simulink model "dx_hand_model_rai3"  (R2017b)
settings: Solver=ode3  StartTime=0.0  StopTime=inf  FixedStep=0.01  RelTol=1e-3  EnableMultiTasking=on
InitFcn:
  | cutFreq = 0.1; % T
  | sampleTime = 0.01;
  | filt = tf(1,[cutFreq 1]);
  | filt = c2d(filt,sampleTime);
  | 
  | cutFreq2 = 1;
  | filt2 = tf(1,[cutFreq2 1]);
  | filt2 = c2d(filt2,sampleTime);
  | 
  | update_param = 2;
  | 
  | ampliFactor = 1.60;
  | ampliFactorMiddle = 2.00;
  | ampliFactorDistal = 1;
  | 
  | % Set Hand Address
  | RightHandAddress = '10.24.4.91';
  | Verosim = '10.100.39.22'
  | LeftHandAddress = '10.24.4.90'
  | 
  | max_force = 12; % Newton
model workspace (MAT data in the model file):
  SL_ROS_VariableLengthArrays_MaxSizes : struct (value not decoded)
libraries: robotlib x134, simulink_extras x28, simulink x16, dspnetwork x5, etargetslib x4
(part 4 of 19)

== system dx_hand_model_rai3/Send to Schunk/Signal Conditioning/Subsystem1 ==
  in_dis_in : Inport
  in_prox_in : Inport  Port=2
  Constant : Constant  Value=0  OutDataTypeStr=single
  Get Parameter3 : robotlib/Get Parameter  SourceLibraryInfo=This block requires Robotics System Toolbox  ParameterSource=Specify your own  ParameterName=/hand_exo/index/enable  ParameterType=double  ParameterMaxArrayLength=16  ParameterInitialValue=1.0  SampleTime=update_param  ShowErrorCodeOutput=on  ModelName=dx_hand_model_rai3  BlockId=ParamGet_dx_hand_model_rai3_2736
      settings: SourceProductName=Robotics System Toolbox  SourceProductBaseCode=RO
  Rate Transition : RateTransition
  Switch : Switch  Criteria=u2 > Threshold
  Switch1 : Switch  Criteria=u2 > Threshold
  in_dis_o : Outport
  in_prox_o : Outport  Port=2
  wires:
  Get Parameter3/1 -> Rate Transition/1
  Constant/1 -> Switch1/3, Switch/3
  in_dis_in/1 -> Switch1/1
  Switch1/1 -> in_dis_o/1
  Switch/1 -> in_prox_o/1
  Rate Transition/1 -> Switch1/2, Switch/2
  in_prox_in/1 -> Switch/1

== system dx_hand_model_rai3/Send to Schunk/Signal Conditioning/Subsystem2 ==
  m_dis_in : Inport
  m_prox_in : Inport  Port=2
  Constant : Constant  Value=0  OutDataTypeStr=single
  Display : Display
  Get Parameter3 : robotlib/Get Parameter  SourceLibraryInfo=This block requires Robotics System Toolbox  ParameterSource=Specify your own  ParameterName=/hand_exo/middle/enable  ParameterType=double  ParameterMaxArrayLength=16  ParameterInitialValue=1.0  SampleTime=update_param  ShowErrorCodeOutput=on  ModelName=dx_hand_model_rai3  BlockId=ParamGet_dx_hand_model_rai3_2745
      settings: SourceProductName=Robotics System Toolbox  SourceProductBaseCode=RO
  Rate Transition : RateTransition
  Switch : Switch  Criteria=u2 > Threshold
  Switch1 : Switch  Criteria=u2 > Threshold
  m_dis_o : Outport
  m_prox_o : Outport  Port=2
  wires:
  Get Parameter3/1 -> Rate Transition/1
  Constant/1 -> Switch1/3, Switch/3
  m_dis_in/1 -> Display/1, Switch1/1
  m_prox_in/1 -> Switch/1
  Switch1/1 -> m_dis_o/1
  Switch/1 -> m_prox_o/1
  Rate Transition/1 -> Switch1/2, Switch/2

== system dx_hand_model_rai3/Send to Schunk/Signal Conditioning/Subsystem3 ==
  r_in : Inport
  Constant : Constant  Value=0.0  OutDataTypeStr=single
  Get Parameter3 : robotlib/Get Parameter  SourceLibraryInfo=This block requires Robotics System Toolbox  ParameterSource=Specify your own  ParameterName=/hand_exo/ring/enable  ParameterType=double  ParameterMaxArrayLength=16  ParameterInitialValue=-1.0  SampleTime=update_param  ShowErrorCodeOutput=on  ModelName=dx_hand_model_rai3  BlockId=ParamGet_dx_hand_model_rai3_2754
      settings: SourceProductName=Robotics System Toolbox  SourceProductBaseCode=RO
  Rate Transition : RateTransition
  Switch1 : Switch  Criteria=u2 > Threshold
  r_o : Outport
  wires:
  Get Parameter3/1 -> Rate Transition/1
  Constant/1 -> Switch1/3
  r_in/1 -> Switch1/1
  Switch1/1 -> r_o/1
  Rate Transition/1 -> Switch1/2

== system dx_hand_model_rai3/Send to Schunk/Signal Conditioning/Subsystem4 ==
  p_in : Inport
  Constant : Constant  Value=0.0  OutDataTypeStr=single
  Get Parameter3 : robotlib/Get Parameter  SourceLibraryInfo=This block requires Robotics System Toolbox  ParameterSource=Specify your own  ParameterName=/hand_exo/pinky/enable  ParameterType=double  ParameterMaxArrayLength=16  ParameterInitialValue=-1.0  SampleTime=update_param  ShowErrorCodeOutput=on  ModelName=dx_hand_model_rai3  BlockId=ParamGet_dx_hand_model_rai3_2762
      settings: SourceProductName=Robotics System Toolbox  SourceProductBaseCode=RO
  Rate Transition : RateTransition
  Switch1 : Switch  Criteria=u2 > Threshold
  p_o : Outport
  wires:
  Get Parameter3/1 -> Rate Transition/1
  Constant/1 -> Switch1/3
  p_in/1 -> Switch1/1
  Switch1/1 -> p_o/1
  Rate Transition/1 -> Switch1/2

== system dx_hand_model_rai3/Send to Schunk/Signal Conditioning/Subsystem5 ==
  s_in : Inport
  Constant : Constant  Value=0.20  OutDataTypeStr=single
  Get Parameter3 : robotlib/Get Parameter  SourceLibraryInfo=This block requires Robotics System Toolbox  ParameterSource=Specify your own  ParameterName=/hand_exo/spread/enable  ParameterType=double  ParameterMaxArrayLength=16  ParameterInitialValue=-1.0  SampleTime=update_param  ShowErrorCodeOutput=on  ModelName=dx_hand_model_rai3  BlockId=ParamGet_dx_hand_model_rai3_2768
      settings: SourceProductName=Robotics System Toolbox  SourceProductBaseCode=RO
  Rate Transition : RateTransition
  Switch1 : Switch  Criteria=u2 > Threshold
  s_o : Outport
  wires:
  Get Parameter3/1 -> Rate Transition/1
  Constant/1 -> Switch1/3
  s_in/1 -> Switch1/1
  Switch1/1 -> s_o/1
  Rate Transition/1 -> Switch1/2

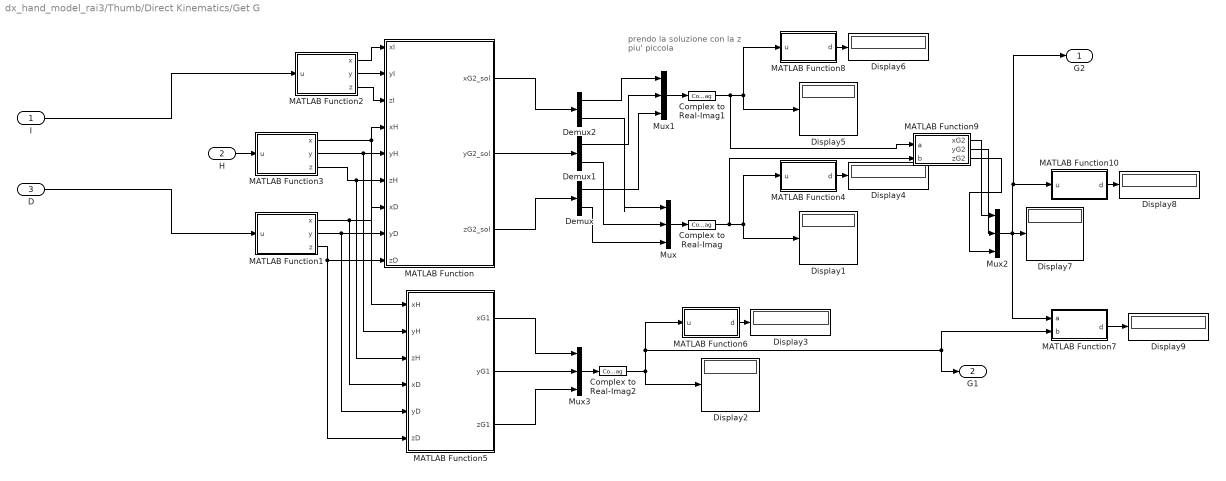
== system dx_hand_model_rai3/Thumb/Direct Kinematics/Get G ==
  note: prendo la soluzione
      | con la z piu' piccola
  I : Inport
  H : Inport  Port=2
  D : Inport  Port=3
  Complex to Real-Imag : ComplexToRealImag  Output=Real
  Complex to Real-Imag1 : ComplexToRealImag  Output=Real
  Complex to Real-Imag2 : ComplexToRealImag  Output=Real
  Demux : Demux  Outputs=2
  Demux1 : Demux  Outputs=2
  Demux2 : Demux  Outputs=2
  Display{1..9} (9 alike) : Display
  MATLAB Function : MATLAB Function  TreatAsAtomicUnit=on
  MATLAB Function1 : MATLAB Function  TreatAsAtomicUnit=on
  MATLAB Function10 : MATLAB Function  TreatAsAtomicUnit=on
  MATLAB Function2 : MATLAB Function  TreatAsAtomicUnit=on
  MATLAB Function3 : MATLAB Function  TreatAsAtomicUnit=on
  MATLAB Function4 : MATLAB Function  TreatAsAtomicUnit=on
  MATLAB Function5 : MATLAB Function  TreatAsAtomicUnit=on
  MATLAB Function6 : MATLAB Function  TreatAsAtomicUnit=on
  MATLAB Function7 : MATLAB Function  TreatAsAtomicUnit=on
  MATLAB Function8 : MATLAB Function  TreatAsAtomicUnit=on
  MATLAB Function9 : MATLAB Function  TreatAsAtomicUnit=on
  Mux{,1..3} (4 alike) : Mux  Inputs=3
  G2 : Outport
  G1 : Outport  Port=2
  wires:
  MATLAB Function1/2(y) -> MATLAB Function/8(yD), MATLAB Function5/5(yD)
  H/1 -> MATLAB Function3/1(u)
  MATLAB Function3/1(x) -> MATLAB Function5/1(xH), MATLAB Function/4(xH)
  MATLAB Function2/1(x) -> MATLAB Function/1(xI)
  D/1 -> MATLAB Function1/1(u)
  MATLAB Function/1(xG2_sol) -> Demux2/1
  Complex to Real-Imag1/1 -> MATLAB Function9/1(a), Display5/1, MATLAB Function8/1(u)
  Demux/2 -> Mux/3
  MATLAB Function10/1(d) -> Display8/1
  MATLAB Function/3(zG2_sol) -> Demux/1
  MATLAB Function2/3(z) -> MATLAB Function/3(zI)
  MATLAB Function2/2(y) -> MATLAB Function/2(yI)
  MATLAB Function9/3(zG2) -> Mux2/3
  Demux2/1 -> Mux1/1
  MATLAB Function1/3(z) -> MATLAB Function5/6(zD), MATLAB Function/9(zD)
  MATLAB Function9/1(xG2) -> Mux2/1
  Demux1/1 -> Mux1/2
  MATLAB Function1/1(x) -> MATLAB Function/7(xD), MATLAB Function5/4(xD)
  Complex to Real-Imag/1 -> MATLAB Function9/2(b), Display1/1, MATLAB Function4/1(u)
  Demux2/2 -> Mux/1
  MATLAB Function9/2(yG2) -> Mux2/2
  I/1 -> MATLAB Function2/1(u)
  Demux/1 -> Mux1/3
  Mux1/1 -> Complex to Real-Imag1/1
  Mux/1 -> Complex to Real-Imag/1
  MATLAB Function3/2(y) -> MATLAB Function5/2(yH), MATLAB Function/5(yH)
  MATLAB Function4/1(d) -> Display4/1
  MATLAB Function3/3(z) -> MATLAB Function/6(zH), MATLAB Function5/3(zH)
  Demux1/2 -> Mux/2
  MATLAB Function/2(yG2_sol) -> Demux1/1
  MATLAB Function8/1(d) -> Display6/1
  Mux3/1 -> Complex to Real-Imag2/1
  MATLAB Function5/2(yG1) -> Mux3/2
  MATLAB Function5/1(xG1) -> Mux3/1
  MATLAB Function5/3(zG1) -> Mux3/3
  MATLAB Function6/1(d) -> Display3/1
  Complex to Real-Imag2/1 -> Display2/1, G1/1, MATLAB Function7/2(b), MATLAB Function6/1(u)
  Mux2/1 -> MATLAB Function7/1(a), G2/1, MATLAB Function10/1(u), Display7/1
  MATLAB Function7/1(d) -> Display9/1

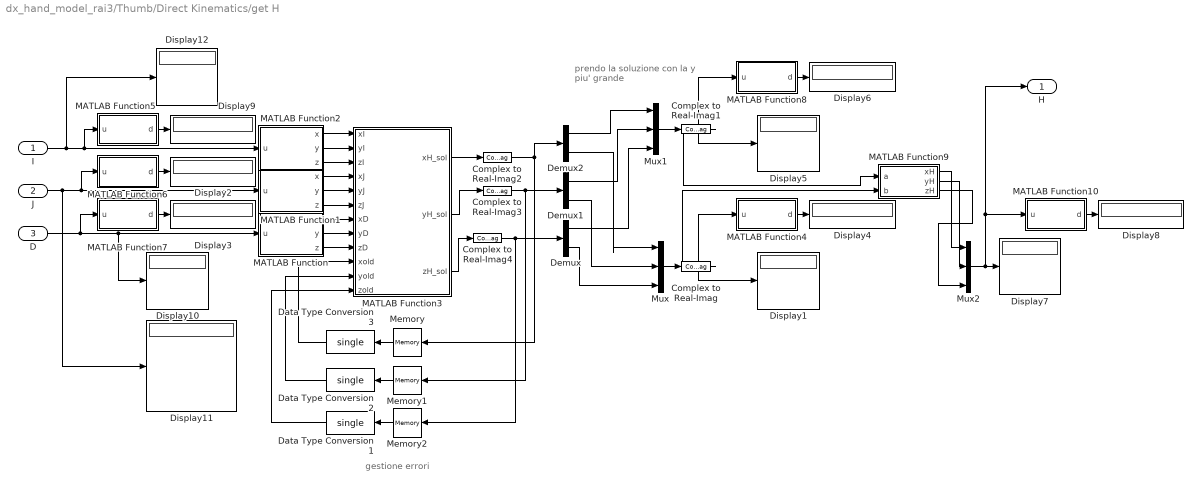
== system dx_hand_model_rai3/Thumb/Direct Kinematics/get H ==
  note: prendo la soluzione
      | con la y piu' grande
  note: gestione errori
  I : Inport
  J : Inport  Port=2
  D : Inport  Port=3
  Complex to Real-Imag{,1..4} (5 alike) : ComplexToRealImag  Output=Real
  Data Type Conversion1 : DataTypeConversion  OutDataTypeStr=single
  Data Type Conversion2 : DataTypeConversion  OutDataTypeStr=single
  Data Type Conversion3 : DataTypeConversion  OutDataTypeStr=single
  Demux : Demux  Outputs=2
  Demux1 : Demux  Outputs=2
  Demux2 : Demux  Outputs=2
  Display{1..12} (12 alike) : Display
  MATLAB Function : MATLAB Function  TreatAsAtomicUnit=on
  MATLAB Function1 : MATLAB Function  TreatAsAtomicUnit=on
  MATLAB Function10 : MATLAB Function  TreatAsAtomicUnit=on
  MATLAB Function2 : MATLAB Function  TreatAsAtomicUnit=on
  MATLAB Function3 : MATLAB Function  TreatAsAtomicUnit=on
  MATLAB Function4 : MATLAB Function  TreatAsAtomicUnit=on
  MATLAB Function5 : MATLAB Function  TreatAsAtomicUnit=on
  MATLAB Function6 : MATLAB Function  TreatAsAtomicUnit=on
  MATLAB Function7 : MATLAB Function  TreatAsAtomicUnit=on
  MATLAB Function8 : MATLAB Function  TreatAsAtomicUnit=on
  MATLAB Function9 : MATLAB Function  TreatAsAtomicUnit=on
  Memory : Memory  InitialCondition=[0,0]
  Memory1 : Memory  InitialCondition=[0,0]
  Memory2 : Memory  InitialCondition=[0,0]
  Mux : Mux  Inputs=3
  Mux1 : Mux  Inputs=3
  Mux2 : Mux  Inputs=3
  H : Outport
  wires:
  MATLAB Function3/1(xH_sol) -> Complex to Real-Imag2/1
  MATLAB Function3/2(yH_sol) -> Complex to Real-Imag3/1
  MATLAB Function9/2(yH) -> Mux2/2
  MATLAB Function9/1(xH) -> Mux2/1
  MATLAB Function4/1(d) -> Display4/1
  Mux2/1 -> H/1, MATLAB Function10/1(u), Display7/1
  Demux2/2 -> Mux/1
  MATLAB Function8/1(d) -> Display6/1
  MATLAB Function6/1(d) -> Display2/1
  MATLAB Function5/1(d) -> Display9/1
  MATLAB Function9/3(zH) -> Mux2/3
  Demux/2 -> Mux/3
  Complex to Real-Imag1/1 -> MATLAB Function9/1(a), Display5/1, MATLAB Function8/1(u)
  Complex to Real-Imag/1 -> MATLAB Function9/2(b), Display1/1, MATLAB Function4/1(u)
  MATLAB Function7/1(d) -> Display3/1
  Demux1/1 -> Mux1/2
  Mux/1 -> Complex to Real-Imag/1
  MATLAB Function10/1(d) -> Display8/1
  Demux2/1 -> Mux1/1
  Demux/1 -> Mux1/3
  MATLAB Function2/2(y) -> MATLAB Function3/2(yI)
  MATLAB Function2/1(x) -> MATLAB Function3/1(xI)
  Demux1/2 -> Mux/2
  MATLAB Function/1(x) -> MATLAB Function3/7(xD)
  D/1 -> MATLAB Function7/1(u), Display10/1, MATLAB Function/1(u)
  MATLAB Function/3(z) -> MATLAB Function3/9(zD)
  MATLAB Function/2(y) -> MATLAB Function3/8(yD)
  MATLAB Function1/1(x) -> MATLAB Function3/4(xJ)
  MATLAB Function1/3(z) -> MATLAB Function3/6(zJ)
  I/1 -> Display12/1, MATLAB Function5/1(u), MATLAB Function2/1(u)
  J/1 -> Display11/1, MATLAB Function6/1(u), MATLAB Function1/1(u)
  MATLAB Function1/2(y) -> MATLAB Function3/5(yJ)
  MATLAB Function2/3(z) -> MATLAB Function3/3(zI)
  Mux1/1 -> Complex to Real-Imag1/1
  MATLAB Function3/3(zH_sol) -> Complex to Real-Imag4/1
  Memory/1 -> Data Type Conversion3/1
  Memory1/1 -> Data Type Conversion2/1
  Memory2/1 -> Data Type Conversion1/1
  Data Type Conversion1/1 -> MATLAB Function3/12(zold)
  Data Type Conversion2/1 -> MATLAB Function3/11(yold)
  Data Type Conversion3/1 -> MATLAB Function3/10(xold)
  Complex to Real-Imag2/1 -> Demux2/1, Memory/1
  Complex to Real-Imag3/1 -> Memory1/1, Demux1/1
  Complex to Real-Imag4/1 -> Memory2/1, Demux/1

== system dx_hand_model_rai3/Thumb/Force Feedback/Active ==
  in : Inport
  Constant : Constant  Value=0  OutDataTypeStr=single
  Data Type Conversion1 : DataTypeConversion  OutDataTypeStr=single
  Get Parameter3 : robotlib/Get Parameter  SourceLibraryInfo=This block requires Robotics System Toolbox  ParameterSource=Specify your own  ParameterName=/hand_exo/thumb/modes/ff_active  ParameterType=double  ParameterMaxArrayLength=16  ParameterInitialValue=1.0  SampleTime=update_param  ShowErrorCodeOutput=off  ModelName=dx_hand_model_rai3  BlockId=ParamGet_dx_hand_model_rai3_4863
      settings: SourceProductName=Robotics System Toolbox  SourceProductBaseCode=RO
  Rate Transition : RateTransition
  Switch : Switch  Criteria=u2 > Threshold
  out : Outport
  wires:
  Switch/1 -> out/1
  Data Type Conversion1/1 -> Switch/2
  Rate Transition/1 -> Data Type Conversion1/1
  Get Parameter3/1 -> Rate Transition/1
  in/1 -> Switch/1
  Constant/1 -> Switch/3

== system dx_hand_model_rai3/Thumb/Force Feedback/g1 ==
  in : Inport
  Data Type Conversion1 : DataTypeConversion  OutDataTypeStr=single
  Get Parameter3 : robotlib/Get Parameter  SourceLibraryInfo=This block requires Robotics System Toolbox  ParameterSource=Specify your own  ParameterName=/hand_exo/thumb/gain/g1  ParameterType=double  ParameterMaxArrayLength=16  ParameterInitialValue=3.5  SampleTime=update_param  ShowErrorCodeOutput=on  ModelName=dx_hand_model_rai3  BlockId=ParamGet_dx_hand_model_rai3_3828
      settings: SourceProductName=Robotics System Toolbox  SourceProductBaseCode=RO
  Product : Product
  Rate Transition : RateTransition
  "out " : Outport
  wires:
  Get Parameter3/1 -> Rate Transition/1
  Rate Transition/1 -> Data Type Conversion1/1
  Data Type Conversion1/1 -> Product/2
  Product/1 -> "out "/1
  in/1 -> Product/1

== system dx_hand_model_rai3/Thumb/Get ADC Values/Angular Potentiometer 1 ==
  ADC : Inport
  Constant : Constant  Value=0  OutDataTypeStr=single
  Constant1 : Constant  Value=420  OutDataTypeStr=single
  Data Type Conversion1 : DataTypeConversion  OutDataTypeStr=single
  Data Type Conversion2 : DataTypeConversion  OutDataTypeStr=double
  Display : Display
  Display1 : Display
  Display2 : Display
  Gain Aggiustato : Gain  Gain=330*pi/(1024*180)
  Get Parameter3 : robotlib/Get Parameter  SourceLibraryInfo=This block requires Robotics System Toolbox  ParameterSource=Specify your own  ParameterName=/hand_exo/thumb/calibration/set1  ParameterType=double  ParameterMaxArrayLength=16  ParameterInitialValue=381  SampleTime=update_param  ShowErrorCodeOutput=on  ModelName=dx_hand_model_rai3  BlockId=ParamGet_dx_hand_model_rai3_2962
      settings: SourceProductName=Robotics System Toolbox  SourceProductBaseCode=RO
  Manual Switch : ManualSwitch
  Radians to Degrees : simulink_extras/Transformations/Radians to Degrees
  Rate Transition : RateTransition
  Set Parameter : robotlib/Set Parameter  SourceLibraryInfo=This block requires Robotics System Toolbox  ParameterSource=Specify your own  ParameterName=/hand_exo/thumb/calibration/get1  ParameterType=double  ModelName=dx_hand_model_rai3  BlockId=ParamSet_dx_hand_model_rai3_2966
      settings: SourceProductName=Robotics System Toolbox  SourceProductBaseCode=RO
  Sum1 : Sum  Inputs=|+-
  Sum2 : Sum  Inputs=|+-
  Deg : Outport
  Rad : Outport  Port=2
  wires:
  ADC/1 -> Data Type Conversion2/1, Sum2/1
  Radians to Degrees/1 -> Display1/1, Deg/1
  Gain Aggiustato/1 -> Display/1, Sum1/1
  Sum1/1 -> Radians to Degrees/1, Rad/1
  Constant/1 -> Sum1/2
  Sum2/1 -> Gain Aggiustato/1
  Get Parameter3/1 -> Rate Transition/1
  Data Type Conversion2/1 -> Set Parameter/1, Display2/1
  Rate Transition/1 -> Data Type Conversion1/1
  Data Type Conversion1/1 -> Manual Switch/1
  Manual Switch/1 -> Sum2/2
  Constant1/1 -> Manual Switch/2

== system dx_hand_model_rai3/Thumb/Get ADC Values/Angular Potentiometer 2 ==
  ADC : Inport
  Constant : Constant  Value=0  OutDataTypeStr=single
  Constant1 : Constant  Value=529  OutDataTypeStr=single
  Data Type Conversion1 : DataTypeConversion  OutDataTypeStr=single
  Data Type Conversion2 : DataTypeConversion  OutDataTypeStr=double
  Display : Display
  Display1 : Display
  Display2 : Display
  Gain Aggiustato : Gain  Gain=330*pi/(1024*180)
  Get Parameter3 : robotlib/Get Parameter  SourceLibraryInfo=This block requires Robotics System Toolbox  ParameterSource=Specify your own  ParameterName=/hand_exo/thumb/calibration/set2  ParameterType=double  ParameterMaxArrayLength=16  ParameterInitialValue=529  SampleTime=update_param  ShowErrorCodeOutput=on  ModelName=dx_hand_model_rai3  BlockId=ParamGet_dx_hand_model_rai3_3019
      settings: SourceProductName=Robotics System Toolbox  SourceProductBaseCode=RO
  Manual Switch : ManualSwitch
  Radians to Degrees : simulink_extras/Transformations/Radians to Degrees
  Rate Transition : RateTransition
  Set Parameter : robotlib/Set Parameter  SourceLibraryInfo=This block requires Robotics System Toolbox  ParameterSource=Specify your own  ParameterName=/hand_exo/thumb/calibration/get2  ParameterType=double  ModelName=dx_hand_model_rai3  BlockId=ParamSet_dx_hand_model_rai3_3023
      settings: SourceProductName=Robotics System Toolbox  SourceProductBaseCode=RO
  Sum1 : Sum  Inputs=|+-
  Sum2 : Sum  Inputs=|+-
  Deg : Outport
  Rad : Outport  Port=2
  wires:
  ADC/1 -> Data Type Conversion2/1, Sum2/1
  Radians to Degrees/1 -> Display1/1, Deg/1
  Gain Aggiustato/1 -> Display/1, Sum1/1
  Sum1/1 -> Radians to Degrees/1, Rad/1
  Constant/1 -> Sum1/2
  Sum2/1 -> Gain Aggiustato/1
  Get Parameter3/1 -> Rate Transition/1
  Data Type Conversion2/1 -> Set Parameter/1, Display2/1
  Rate Transition/1 -> Data Type Conversion1/1
  Data Type Conversion1/1 -> Manual Switch/1
  Manual Switch/1 -> Sum2/2
  Constant1/1 -> Manual Switch/2

== system dx_hand_model_rai3/Thumb/Get ADC Values/Angular Potentiometer 3 ==
  ADC : Inport
  Constant : Constant  Value=0  OutDataTypeStr=single
  Constant1 : Constant  Value=576  OutDataTypeStr=single
  Data Type Conversion1 : DataTypeConversion  OutDataTypeStr=single
  Data Type Conversion2 : DataTypeConversion  OutDataTypeStr=double
  Display : Display
  Display1 : Display
  Display2 : Display
  Gain Aggiustato : Gain  Gain=330*pi/(1024*180)
  Get Parameter3 : robotlib/Get Parameter  SourceLibraryInfo=This block requires Robotics System Toolbox  ParameterSource=Specify your own  ParameterName=/hand_exo/thumb/calibration/set3  ParameterType=double  ParameterMaxArrayLength=16  ParameterInitialValue=576  SampleTime=update_param  ShowErrorCodeOutput=on  ModelName=dx_hand_model_rai3  BlockId=ParamGet_dx_hand_model_rai3_3038
      settings: SourceProductName=Robotics System Toolbox  SourceProductBaseCode=RO
  Manual Switch : ManualSwitch
  Radians to Degrees : simulink_extras/Transformations/Radians to Degrees
  Rate Transition : RateTransition
  Set Parameter : robotlib/Set Parameter  SourceLibraryInfo=This block requires Robotics System Toolbox  ParameterSource=Specify your own  ParameterName=/hand_exo/thumb/calibration/get3  ParameterType=double  ModelName=dx_hand_model_rai3  BlockId=ParamSet_dx_hand_model_rai3_3042
      settings: SourceProductName=Robotics System Toolbox  SourceProductBaseCode=RO
  Sum1 : Sum  Inputs=|+-
  Sum2 : Sum  Inputs=|+-
  Deg : Outport
  Rad : Outport  Port=2
  wires:
  ADC/1 -> Data Type Conversion2/1, Sum2/1
  Radians to Degrees/1 -> Display1/1, Deg/1
  Gain Aggiustato/1 -> Display/1, Sum1/1
  Sum1/1 -> Radians to Degrees/1, Rad/1
  Constant/1 -> Sum1/2
  Sum2/1 -> Gain Aggiustato/1
  Get Parameter3/1 -> Rate Transition/1
  Data Type Conversion2/1 -> Set Parameter/1, Display2/1
  Rate Transition/1 -> Data Type Conversion1/1
  Data Type Conversion1/1 -> Manual Switch/1
  Manual Switch/1 -> Sum2/2
  Constant1/1 -> Manual Switch/2

== system dx_hand_model_rai3/Thumb/Get ADC Values/Angular Potentiometer 4 ==
  ADC : Inport
  Constant2 : Constant  Value=517  OutDataTypeStr=single
  Data Type Conversion1 : DataTypeConversion  OutDataTypeStr=single
  Data Type Conversion2 : DataTypeConversion  OutDataTypeStr=double
  Display : Display
  Display1 : Display
  Display3 : Display
  Gain Aggiustato : Gain  Gain=330*pi/(1024*180)
  Get Parameter3 : robotlib/Get Parameter  SourceLibraryInfo=This block requires Robotics System Toolbox  ParameterSource=Specify your own  ParameterName=/hand_exo/thumb/calibration/set4  ParameterType=double  ParameterMaxArrayLength=16  ParameterInitialValue=517.0  SampleTime=update_param  ShowErrorCodeOutput=on  ModelName=dx_hand_model_rai3  BlockId=ParamGet_dx_hand_model_rai3_4259
      settings: SourceProductName=Robotics System Toolbox  SourceProductBaseCode=RO
  Manual Switch : ManualSwitch
  Radians to Degrees : simulink_extras/Transformations/Radians to Degrees
  Rate Transition : RateTransition
  Set Parameter : robotlib/Set Parameter  SourceLibraryInfo=This block requires Robotics System Toolbox  ParameterSource=Specify your own  ParameterName=/hand_exo/thumb/calibration/get4  ParameterType=double  ModelName=dx_hand_model_rai3  BlockId=ParamSet_dx_hand_model_rai3_4262
      settings: SourceProductName=Robotics System Toolbox  SourceProductBaseCode=RO
  Sign : Gain  Gain=-1
  Sum2 : Sum  Inputs=|+-
  Deg : Outport
  Rad : Outport  Port=2
  wires:
  Radians to Degrees/1 -> Display1/1, Deg/1
  ADC/1 -> Sum2/1, Data Type Conversion2/1
  Gain Aggiustato/1 -> Sign/1, Display/1
  Sign/1 -> Radians to Degrees/1, Rad/1
  Sum2/1 -> Gain Aggiustato/1
  Manual Switch/1 -> Sum2/2
  Get Parameter3/1 -> Rate Transition/1
  Data Type Conversion2/1 -> Set Parameter/1, Display3/1
  Rate Transition/1 -> Data Type Conversion1/1
  Data Type Conversion1/1 -> Manual Switch/1
  Constant2/1 -> Manual Switch/2

== system dx_hand_model_rai3/Thumb/Get ADC Values/Angular Potentiometer 5 ==
  ADC : Inport
  Constant2 : Constant  Value=579  OutDataTypeStr=single
  Data Type Conversion1 : DataTypeConversion  OutDataTypeStr=single
  Data Type Conversion2 : DataTypeConversion  OutDataTypeStr=double
  Display : Display
  Display1 : Display
  Display3 : Display
  Gain Aggiustato : Gain  Gain=330*pi/(1024*180)
  Get Parameter3 : robotlib/Get Parameter  SourceLibraryInfo=This block requires Robotics System Toolbox  ParameterSource=Specify your own  ParameterName=/hand_exo/thumb/calibration/set5  ParameterType=double  ParameterMaxArrayLength=16  ParameterInitialValue=579.0  SampleTime=update_param  ShowErrorCodeOutput=on  ModelName=dx_hand_model_rai3  BlockId=ParamGet_dx_hand_model_rai3_4267
      settings: SourceProductName=Robotics System Toolbox  SourceProductBaseCode=RO
  Manual Switch : ManualSwitch
  Radians to Degrees : simulink_extras/Transformations/Radians to Degrees
  Rate Transition : RateTransition
  Set Parameter : robotlib/Set Parameter  SourceLibraryInfo=This block requires Robotics System Toolbox  ParameterSource=Specify your own  ParameterName=/hand_exo/thumb/calibration/get5  ParameterType=double  ModelName=dx_hand_model_rai3  BlockId=ParamSet_dx_hand_model_rai3_4270
      settings: SourceProductName=Robotics System Toolbox  SourceProductBaseCode=RO
  Sign : Gain
  Sum2 : Sum  Inputs=|+-
  Deg : Outport
  Rad : Outport  Port=2
  wires:
  Radians to Degrees/1 -> Display1/1, Deg/1
  Gain Aggiustato/1 -> Sign/1, Display/1
  Sign/1 -> Radians to Degrees/1, Rad/1
  Sum2/1 -> Gain Aggiustato/1
  ADC/1 -> Data Type Conversion2/1, Sum2/1
  Manual Switch/1 -> Sum2/2
  Get Parameter3/1 -> Rate Transition/1
  Constant2/1 -> Manual Switch/2
  Data Type Conversion2/1 -> Set Parameter/1, Display3/1
  Rate Transition/1 -> Data Type Conversion1/1
  Data Type Conversion1/1 -> Manual Switch/1

== system dx_hand_model_rai3/Thumb/Get_from_ROS_param/Subsystem ==
  In1 : Inport
  Data Type Conversion1 : DataTypeConversion  OutDataTypeStr=single
  Rate Transition : RateTransition  InitialCondition=-10.0
  Out1 : Outport
  wires:
  Data Type Conversion1/1 -> Out1/1
  In1/1 -> Rate Transition/1
  Rate Transition/1 -> Data Type Conversion1/1

== system dx_hand_model_rai3/Thumb/Get_from_ROS_param/Subsystem1 ==
  In1 : Inport
  Data Type Conversion1 : DataTypeConversion  OutDataTypeStr=single
  Rate Transition : RateTransition  InitialCondition=0.0
  Out1 : Outport
  wires:
  Data Type Conversion1/1 -> Out1/1
  In1/1 -> Rate Transition/1
  Rate Transition/1 -> Data Type Conversion1/1

== system dx_hand_model_rai3/Thumb/Get_from_ROS_param/Subsystem2 ==
  In1 : Inport
  Data Type Conversion1 : DataTypeConversion  OutDataTypeStr=single
  Rate Transition : RateTransition  InitialCondition=-32.0
  Out1 : Outport
  wires:
  Data Type Conversion1/1 -> Out1/1
  In1/1 -> Rate Transition/1
  Rate Transition/1 -> Data Type Conversion1/1

== system dx_hand_model_rai3/Thumb/Get_from_ROS_param/Subsystem3 ==
  In1 : Inport
  Data Type Conversion1 : DataTypeConversion  OutDataTypeStr=single
  Rate Transition : RateTransition  InitialCondition=20.0
  Out1 : Outport
  wires:
  Data Type Conversion1/1 -> Out1/1
  In1/1 -> Rate Transition/1
  Rate Transition/1 -> Data Type Conversion1/1

== system dx_hand_model_rai3/Thumb/Get_from_ROS_param/Subsystem4 ==
  In1 : Inport
  Data Type Conversion1 : DataTypeConversion  OutDataTypeStr=single
  Rate Transition : RateTransition  InitialCondition=50.0
  Out1 : Outport
  wires:
  Data Type Conversion1/1 -> Out1/1
  In1/1 -> Rate Transition/1
  Rate Transition/1 -> Data Type Conversion1/1

== system dx_hand_model_rai3/Thumb/Get_from_ROS_param/Subsystem5 ==
  In1 : Inport
  Data Type Conversion1 : DataTypeConversion  OutDataTypeStr=single
  Rate Transition : RateTransition  InitialCondition=20.0
  Out1 : Outport
  wires:
  Data Type Conversion1/1 -> Out1/1
  In1/1 -> Rate Transition/1
  Rate Transition/1 -> Data Type Conversion1/1

== system dx_hand_model_rai3/Thumb/Get_from_ROS_param/Subsystem6 ==
  In1 : Inport
  Data Type Conversion1 : DataTypeConversion  OutDataTypeStr=single
  Rate Transition : RateTransition  InitialCondition=50.0
  Out1 : Outport
  wires:
  Data Type Conversion1/1 -> Out1/1
  In1/1 -> Rate Transition/1
  Rate Transition/1 -> Data Type Conversion1/1

== system dx_hand_model_rai3/Thumb/Old Stuff/calibration ==
  In1 : Inport
  Constant2 : Constant  Value=540  OutDataTypeStr=single
  Constant3 : Constant  Value=540  OutDataTypeStr=single
  Display4 : Display
  Subsystem : Subsystem
  Sum2 : Sum  Inputs=|++
  Switch : Switch  Criteria=u2 > Threshold
  Out1 : Outport
  wires:
  [CalibrationSignal] -> Switch/2
  Subsystem/1(Out1) -> Switch/3
  Constant3/1 -> Sum2/1
  [CalibrationSignal] -> Subsystem/Enable
  Constant2/1 -> Switch/1
  Sum2/1 -> Display4/1, Subsystem/1(In1)
  In1/1 -> Sum2/2
  Switch/1 -> Out1/1

== system dx_hand_model_rai3/Thumb/Old Stuff/calibration1 ==
  In1 : Inport
  Subsystem1 : Subsystem
  Out1 : Outport
  wires:
  [CalibrationSignal] -> Subsystem1/Enable
  In1/1 -> Subsystem1/1(In1)
  Subsystem1/1(Out1) -> Out1/1

== system dx_hand_model_rai3/Thumb/Study Gravity Compensation/Subsystem2 ==
  In1 : Inport
  In2 : Inport  Port=2
  Enable : EnablePort
  Data Type Conversion1 : DataTypeConversion  OutDataTypeStr=double
  Mux : Mux  Inputs=2
  To File : ToFile  Filename=thumb_force.mat  MatrixName=forza_gravita
  wires:
  In1/1 -> Mux/1
  Mux/1 -> Data Type Conversion1/1
  In2/1 -> Mux/2
  Data Type Conversion1/1 -> To File/1

== system dx_hand_model_rai3/Thumb/ToSchunk/Subsystem ==
  Data Type Conversion1 : DataTypeConversion  OutDataTypeStr=single
  Get Parameter3 : robotlib/Get Parameter  SourceLibraryInfo=This block requires Robotics System Toolbox  ParameterSource=Specify your own  ParameterName=/hand_exo/thumb/offset/opp  ParameterType=double  ParameterMaxArrayLength=16  ParameterInitialValue=0.5  SampleTime=update_param  ShowErrorCodeOutput=on  ModelName=dx_hand_model_rai3  BlockId=ParamGet_dx_hand_model_rai3_3810
      settings: SourceProductName=Robotics System Toolbox  SourceProductBaseCode=RO
  Rate Transition : RateTransition
  offset : Outport
  wires:
  Get Parameter3/1 -> Rate Transition/1
  Rate Transition/1 -> Data Type Conversion1/1
  Data Type Conversion1/1 -> offset/1

== system dx_hand_model_rai3/Thumb/ToSchunk/Subsystem1 ==
  Data Type Conversion1 : DataTypeConversion  OutDataTypeStr=single
  Get Parameter3 : robotlib/Get Parameter  SourceLibraryInfo=This block requires Robotics System Toolbox  ParameterSource=Specify your own  ParameterName=/hand_exo/thumb/offset/flex  ParameterType=double  ParameterMaxArrayLength=16  ParameterInitialValue=5.0  SampleTime=update_param  ShowErrorCodeOutput=on  ModelName=dx_hand_model_rai3  BlockId=ParamGet_dx_hand_model_rai3_3817
      settings: SourceProductName=Robotics System Toolbox  SourceProductBaseCode=RO
  Rate Transition : RateTransition
  offset : Outport
  wires:
  Get Parameter3/1 -> Rate Transition/1
  Rate Transition/1 -> Data Type Conversion1/1
  Data Type Conversion1/1 -> offset/1

== system dx_hand_model_rai3/Get From Schunk/Get positions/Get Positions/Filter ==
  enable : Inport
  in : Inport  Port=2
  Filt 4 : DiscreteTransferFcn  Numerator=filt2.Numerator{1,1}  Denominator=filt2.Denominator{1,1}  SampleTime=0.01
  Switch : Switch  Criteria=u2 > Threshold
  out : Outport
  wires:
  in/1 -> Switch/3, Filt 4/1
  Switch/1 -> out/1
  Filt 4/1 -> Switch/1
  enable/1 -> Switch/2

== system dx_hand_model_rai3/Get From Schunk/Get positions/Get Positions/Filter1 ==
  enable : Inport
  in : Inport  Port=2
  Filt 4 : DiscreteTransferFcn  Numerator=filt2.Numerator{1,1}  Denominator=filt2.Denominator{1,1}  SampleTime=0.01
  Switch : Switch  Criteria=u2 > Threshold
  out : Outport
  wires:
  in/1 -> Switch/3, Filt 4/1
  Switch/1 -> out/1
  Filt 4/1 -> Switch/1
  enable/1 -> Switch/2

== system dx_hand_model_rai3/Get From Schunk/Get positions/Get Positions/Filter2 ==
  enable : Inport
  in : Inport  Port=2
  Filt 4 : DiscreteTransferFcn  Numerator=filt2.Numerator{1,1}  Denominator=filt2.Denominator{1,1}  SampleTime=0.01
  Switch : Switch  Criteria=u2 > Threshold
  out : Outport
  wires:
  in/1 -> Switch/3, Filt 4/1
  Switch/1 -> out/1
  Filt 4/1 -> Switch/1
  enable/1 -> Switch/2

== system dx_hand_model_rai3/Get From Schunk/Get positions/Get Positions/Filter3 ==
  enable : Inport
  in : Inport  Port=2
  Filt 4 : DiscreteTransferFcn  Numerator=filt2.Numerator{1,1}  Denominator=filt2.Denominator{1,1}  SampleTime=0.01
  Switch : Switch  Criteria=u2 > Threshold
  out : Outport
  wires:
  in/1 -> Switch/3, Filt 4/1
  Switch/1 -> out/1
  Filt 4/1 -> Switch/1
  enable/1 -> Switch/2

== system dx_hand_model_rai3/Get From Schunk/Get positions/Get Positions/Filter4 ==
  enable : Inport
  in : Inport  Port=2
  Filt 4 : DiscreteTransferFcn  Numerator=filt2.Numerator{1,1}  Denominator=filt2.Denominator{1,1}  SampleTime=0.01
  Switch : Switch  Criteria=u2 > Threshold
  out : Outport
  wires:
  in/1 -> Switch/3, Filt 4/1
  Switch/1 -> out/1
  Filt 4/1 -> Switch/1
  enable/1 -> Switch/2

== system dx_hand_model_rai3/Get From Schunk/Get positions/Get Positions/Filter5 ==
  enable : Inport
  in : Inport  Port=2
  Filt 4 : DiscreteTransferFcn  Numerator=filt2.Numerator{1,1}  Denominator=filt2.Denominator{1,1}  SampleTime=0.01
  Switch : Switch  Criteria=u2 > Threshold
  out : Outport
  wires:
  in/1 -> Switch/3, Filt 4/1
  Switch/1 -> out/1
  Filt 4/1 -> Switch/1
  enable/1 -> Switch/2

== system dx_hand_model_rai3/Index Finger/Force/Position Force Basic Architecture/pos_gains//dist ==
  pre_dist : Inport
  Constant : Constant  Value=10  OutDataTypeStr=single
  Data Type Conversion1 : DataTypeConversion  OutDataTypeStr=single
  Data Type Conversion2 : DataTypeConversion  OutDataTypeStr=single
  Get Parameter3 : robotlib/Get Parameter  SourceLibraryInfo=This block requires Robotics System Toolbox  ParameterSource=Specify your own  ParameterName=/hand_exo/index/f_gains/dist  ParameterType=double  ParameterMaxArrayLength=16  ParameterInitialValue=0.0  SampleTime=update_param  ShowErrorCodeOutput=on  ModelName=dx_hand_model_rai3  BlockId=ParamGet_dx_hand_model_rai3_3578
      settings: SourceProductName=Robotics System Toolbox  SourceProductBaseCode=RO
  Manual Switch : ManualSwitch
  Product : Product
  Rate Transition : RateTransition
  post_dist : Outport
  wires:
  Get Parameter3/1 -> Rate Transition/1
  pre_dist/1 -> Product/2
  Product/1 -> Data Type Conversion1/1
  Data Type Conversion1/1 -> post_dist/1
  Rate Transition/1 -> Data Type Conversion2/1
  Constant/1 -> Manual Switch/2
  Data Type Conversion2/1 -> Manual Switch/1
  Manual Switch/1 -> Product/1

== system dx_hand_model_rai3/Index Finger/Force/Position Force Basic Architecture/pos_gains//prox ==
  pre_prox : Inport
  Constant : Constant  Value=-15  OutDataTypeStr=single
  Data Type Conversion1 : DataTypeConversion  OutDataTypeStr=single
  Data Type Conversion2 : DataTypeConversion  OutDataTypeStr=single
  Get Parameter3 : robotlib/Get Parameter  SourceLibraryInfo=This block requires Robotics System Toolbox  ParameterSource=Specify your own  ParameterName=/hand_exo/index/f_gains/prox  ParameterType=double  ParameterMaxArrayLength=16  ParameterInitialValue=-15  SampleTime=update_param  ShowErrorCodeOutput=on  ModelName=dx_hand_model_rai3  BlockId=ParamGet_dx_hand_model_rai3_3588
      settings: SourceProductName=Robotics System Toolbox  SourceProductBaseCode=RO
  Manual Switch : ManualSwitch
  Product : Product
  Rate Transition : RateTransition
  post_prox : Outport
  wires:
  Get Parameter3/1 -> Rate Transition/1
  pre_prox/1 -> Product/2
  Product/1 -> Data Type Conversion1/1
  Data Type Conversion1/1 -> post_prox/1
  Rate Transition/1 -> Data Type Conversion2/1
  Data Type Conversion2/1 -> Manual Switch/1
  Manual Switch/1 -> Product/1
  Constant/1 -> Manual Switch/2

== system dx_hand_model_rai3/Index Finger/Pose Generator/Parametri Dito/Get_from_ROS_param ==
  Get Parameter : robotlib/Get Parameter  SourceLibraryInfo=This block requires Robotics System Toolbox  ParameterSource=Specify your own  ParameterName=/hand_exo/index/offx  ParameterType=double  ParameterMaxArrayLength=16  ParameterInitialValue=0.0  SampleTime=update_param  ShowErrorCodeOutput=on  ModelName=dx_hand_model_rai3  BlockId=ParamGet_dx_hand_model_rai3_2613
      settings: SourceProductName=Robotics System Toolbox  SourceProductBaseCode=RO
  Get Parameter1 : robotlib/Get Parameter  SourceLibraryInfo=This block requires Robotics System Toolbox  ParameterSource=Specify your own  ParameterName=/hand_exo/index/offy  ParameterType=double  ParameterMaxArrayLength=16  ParameterInitialValue=20.0  SampleTime=update_param  ShowErrorCodeOutput=on  ModelName=dx_hand_model_rai3  BlockId=ParamGet_dx_hand_model_rai3_2614
      settings: SourceProductName=Robotics System Toolbox  SourceProductBaseCode=RO
  Get Parameter2 : robotlib/Get Parameter  SourceLibraryInfo=This block requires Robotics System Toolbox  ParameterSource=Specify your own  ParameterName=/hand_exo/index/length  ParameterType=double  ParameterMaxArrayLength=16  ParameterInitialValue=44.0  SampleTime=update_param  ShowErrorCodeOutput=on  ModelName=dx_hand_model_rai3  BlockId=ParamGet_dx_hand_model_rai3_2615
      settings: SourceProductName=Robotics System Toolbox  SourceProductBaseCode=RO
  Get Parameter3 : robotlib/Get Parameter  SourceLibraryInfo=This block requires Robotics System Toolbox  ParameterSource=Specify your own  ParameterName=/hand_exo/index/s  ParameterType=double  ParameterMaxArrayLength=16  ParameterInitialValue=8.5  SampleTime=update_param  ShowErrorCodeOutput=on  ModelName=dx_hand_model_rai3  BlockId=ParamGet_dx_hand_model_rai3_2616
      settings: SourceProductName=Robotics System Toolbox  SourceProductBaseCode=RO
  Get Parameter4 : robotlib/Get Parameter  SourceLibraryInfo=This block requires Robotics System Toolbox  ParameterSource=Specify your own  ParameterName=/hand_exo/index/offa  ParameterType=double  ParameterMaxArrayLength=16  ParameterInitialValue=0  SampleTime=update_param  ShowErrorCodeOutput=on  ModelName=dx_hand_model_rai3  BlockId=ParamGet_dx_hand_model_rai3_2617
      settings: SourceProductName=Robotics System Toolbox  SourceProductBaseCode=RO
  Mux : Mux  Inputs=5
  Terminator{,1..4} (5 alike) : Terminator
  param : Outport
  wires:
  Get Parameter/1 -> Mux/3
  Get Parameter1/1 -> Mux/4
  Get Parameter2/1 -> Mux/2
  Get Parameter4/1 -> Mux/5
  Get Parameter2/2 -> Terminator1/1
  Mux/1 -> param/1
  Get Parameter4/2 -> Terminator4/1
  Get Parameter/2 -> Terminator2/1
  Get Parameter1/2 -> Terminator3/1
  Get Parameter3/1 -> Mux/1
  Get Parameter3/2 -> Terminator/1

== system dx_hand_model_rai3/Index Finger/Pose Generator/Parametri Dito/Hand Written ==
  Antonio1 : Constant  Value="[8.5   44    0    20 0]"
  Indice Legno Misurato : Constant  Value="[11   55    5   25.9]"
  param : Outport
  wires:
  Antonio1/1 -> param/1

== system dx_hand_model_rai3/Middle Finger/Pose Generator/Parametri Dito/Get_from_ROS_param ==
  Get Parameter : robotlib/Get Parameter  SourceLibraryInfo=This block requires Robotics System Toolbox  ParameterSource=Select from ROS network  ParameterName=/hand_exo/middle/offx  ParameterType=double  ParameterMaxArrayLength=16  ParameterInitialValue=0  SampleTime=update_param  ShowErrorCodeOutput=on  ModelName=dx_hand_model_rai3  BlockId=ParamGet_dx_hand_model_rai3_2519
      settings: SourceProductName=Robotics System Toolbox  SourceProductBaseCode=RO
  Get Parameter1 : robotlib/Get Parameter  SourceLibraryInfo=This block requires Robotics System Toolbox  ParameterSource=Specify your own  ParameterName=/hand_exo/middle/offy  ParameterType=double  ParameterMaxArrayLength=16  ParameterInitialValue=23.4  SampleTime=update_param  ShowErrorCodeOutput=on  ModelName=dx_hand_model_rai3  BlockId=ParamGet_dx_hand_model_rai3_2520
      settings: SourceProductName=Robotics System Toolbox  SourceProductBaseCode=RO
  Get Parameter2 : robotlib/Get Parameter  SourceLibraryInfo=This block requires Robotics System Toolbox  ParameterSource=Specify your own  ParameterName=/hand_exo/middle/length  ParameterType=double  ParameterMaxArrayLength=16  ParameterInitialValue=44.8  SampleTime=update_param  ShowErrorCodeOutput=on  ModelName=dx_hand_model_rai3  BlockId=ParamGet_dx_hand_model_rai3_2521
      settings: SourceProductName=Robotics System Toolbox  SourceProductBaseCode=RO
  Get Parameter3 : robotlib/Get Parameter  SourceLibraryInfo=This block requires Robotics System Toolbox  ParameterSource=Specify your own  ParameterName=/hand_exo/middle/s  ParameterType=double  ParameterMaxArrayLength=16  ParameterInitialValue=8.0  SampleTime=update_param  ShowErrorCodeOutput=on  ModelName=dx_hand_model_rai3  BlockId=ParamGet_dx_hand_model_rai3_2522
      settings: SourceProductName=Robotics System Toolbox  SourceProductBaseCode=RO
  Get Parameter4 : robotlib/Get Parameter  SourceLibraryInfo=This block requires Robotics System Toolbox  ParameterSource=Specify your own  ParameterName=/hand_exo/middle/offa  ParameterType=double  ParameterMaxArrayLength=16  ParameterInitialValue=0  SampleTime=update_param  ShowErrorCodeOutput=on  ModelName=dx_hand_model_rai3  BlockId=ParamGet_dx_hand_model_rai3_2523
      settings: SourceProductName=Robotics System Toolbox  SourceProductBaseCode=RO
  Mux : Mux  Inputs=5
  Terminator{,1..4} (5 alike) : Terminator
  param : Outport
  wires:
  Get Parameter/1 -> Mux/3
  Get Parameter1/1 -> Mux/4
  Get Parameter2/1 -> Mux/2
  Get Parameter4/1 -> Mux/5
  Get Parameter2/2 -> Terminator1/1
  Mux/1 -> param/1
  Get Parameter4/2 -> Terminator4/1
  Get Parameter/2 -> Terminator2/1
  Get Parameter1/2 -> Terminator3/1
  Get Parameter3/1 -> Mux/1
  Get Parameter3/2 -> Terminator/1

== system dx_hand_model_rai3/Middle Finger/Pose Generator/Parametri Dito/Hand_written ==
  Antonio : Constant  Value=[ 8, 44.755952819297409619589520899781, 0, 1645979925414585/70368744177664, 0]
  Antonio Stimato : Constant  Value="[10.0000   46.0001    5.0000   17.9112         0]"
  Mano Domenico Stimata : Constant  Value="[9.5248   43.5033         0   10.2567   -1.6252]"
  Mano Legno : Constant  Value="[8   56   6    23 0]"
  Mano Legno Stimata : Constant  Value=[ 8, 60.637566881231091700096944861316, 0, 5166787254901141/281474976710656 0]
  Mano Legno Stimata1 : Constant  Value="[9.9977   51.1548    2.0668   25.1677         0]"
  Mano Legno1 : Constant  Value="[10.8169   54.9796    1.9601   28.8058]"
  Mano Max Reale : Constant  Value=[8 40 0 23 0]
  Mano Max Stimata : Constant  Value=[ 8, 48.37173324617629829549070114942, 0, 6626664510253941/281474976710656, 0]
  Mano Paolo Stimata : Constant  Value="[10.0000   46.0015    1.3696   13.2621         0]"
  Out2 : Outport
  wires:
  Antonio/1 -> Out2/1

== system dx_hand_model_rai3/Middle Finger/Position-Force Architecture/Position Force Basic Architecture/pos_gains//dist ==
  pre_dist : Inport
  Constant : Constant  Value=10  OutDataTypeStr=single
  Data Type Conversion1 : DataTypeConversion  OutDataTypeStr=single
  Data Type Conversion2 : DataTypeConversion  OutDataTypeStr=single
  Get Parameter3 : robotlib/Get Parameter  SourceLibraryInfo=This block requires Robotics System Toolbox  ParameterSource=Specify your own  ParameterName=/hand_exo/middle/f_gains/dist  ParameterType=double  ParameterMaxArrayLength=16  ParameterInitialValue=10  SampleTime=update_param  ShowErrorCodeOutput=on  ModelName=dx_hand_model_rai3  BlockId=ParamGet_dx_hand_model_rai3_2703
      settings: SourceProductName=Robotics System Toolbox  SourceProductBaseCode=RO
  Manual Switch : ManualSwitch
  Product : Product
  Rate Transition : RateTransition
  post_dist : Outport
  wires:
  Get Parameter3/1 -> Rate Transition/1
  pre_dist/1 -> Product/2
  Product/1 -> Data Type Conversion1/1
  Data Type Conversion1/1 -> post_dist/1
  Rate Transition/1 -> Data Type Conversion2/1
  Constant/1 -> Manual Switch/2
  Data Type Conversion2/1 -> Manual Switch/1
  Manual Switch/1 -> Product/1

== system dx_hand_model_rai3/Middle Finger/Position-Force Architecture/Position Force Basic Architecture/pos_gains//prox ==
  pre_prox : Inport
  Constant : Constant  Value=-15  OutDataTypeStr=single
  Data Type Conversion1 : DataTypeConversion  OutDataTypeStr=single
  Data Type Conversion2 : DataTypeConversion  OutDataTypeStr=single
  Get Parameter3 : robotlib/Get Parameter  SourceLibraryInfo=This block requires Robotics System Toolbox  ParameterSource=Specify your own  ParameterName=/hand_exo/middle/f_gains/prox  ParameterType=double  ParameterMaxArrayLength=16  ParameterInitialValue=-15  SampleTime=update_param  ShowErrorCodeOutput=on  ModelName=dx_hand_model_rai3  BlockId=ParamGet_dx_hand_model_rai3_2713
      settings: SourceProductName=Robotics System Toolbox  SourceProductBaseCode=RO
  Manual Switch : ManualSwitch
  Product : Product
  Rate Transition : RateTransition
  post_prox : Outport
  wires:
  Get Parameter3/1 -> Rate Transition/1
  pre_prox/1 -> Product/2
  Product/1 -> Data Type Conversion1/1
  Data Type Conversion1/1 -> post_prox/1
  Rate Transition/1 -> Data Type Conversion2/1
  Data Type Conversion2/1 -> Manual Switch/1
  Manual Switch/1 -> Product/1
  Constant/1 -> Manual Switch/2

== system dx_hand_model_rai3/Pinky Finger/Pose Generator/Parametri Ring/Get_from_ROS_param ==
  Get Parameter : robotlib/Get Parameter  SourceLibraryInfo=This block requires Robotics System Toolbox  ParameterSource=Specify your own  ParameterName=/hand_exo/pinky/offx  ParameterType=double  ParameterMaxArrayLength=16  ParameterInitialValue=0  SampleTime=update_param  ShowErrorCodeOutput=on  ModelName=dx_hand_model_rai3  BlockId=ParamGet_dx_hand_model_rai3_4640
      settings: SourceProductName=Robotics System Toolbox  SourceProductBaseCode=RO
  Get Parameter1 : robotlib/Get Parameter  SourceLibraryInfo=This block requires Robotics System Toolbox  ParameterSource=Specify your own  ParameterName=/hand_exo/pinky/offy  ParameterType=double  ParameterMaxArrayLength=16  ParameterInitialValue=23.4  SampleTime=update_param  ShowErrorCodeOutput=on  ModelName=dx_hand_model_rai3  BlockId=ParamGet_dx_hand_model_rai3_4641
      settings: SourceProductName=Robotics System Toolbox  SourceProductBaseCode=RO
  Get Parameter2 : robotlib/Get Parameter  SourceLibraryInfo=This block requires Robotics System Toolbox  ParameterSource=Specify your own  ParameterName=/hand_exo/pinky/length  ParameterType=double  ParameterMaxArrayLength=16  ParameterInitialValue=44.8  SampleTime=update_param  ShowErrorCodeOutput=on  ModelName=dx_hand_model_rai3  BlockId=ParamGet_dx_hand_model_rai3_4642
      settings: SourceProductName=Robotics System Toolbox  SourceProductBaseCode=RO
  Get Parameter3 : robotlib/Get Parameter  SourceLibraryInfo=This block requires Robotics System Toolbox  ParameterSource=Specify your own  ParameterName=/hand_exo/pinky/s  ParameterType=double  ParameterMaxArrayLength=16  ParameterInitialValue=8.0  SampleTime=update_param  ShowErrorCodeOutput=on  ModelName=dx_hand_model_rai3  BlockId=ParamGet_dx_hand_model_rai3_4643
      settings: SourceProductName=Robotics System Toolbox  SourceProductBaseCode=RO
  Get Parameter4 : robotlib/Get Parameter  SourceLibraryInfo=This block requires Robotics System Toolbox  ParameterSource=Specify your own  ParameterName=/hand_exo/pinky/offa  ParameterType=double  ParameterMaxArrayLength=16  ParameterInitialValue=0  SampleTime=update_param  ShowErrorCodeOutput=on  ModelName=dx_hand_model_rai3  BlockId=ParamGet_dx_hand_model_rai3_4644
      settings: SourceProductName=Robotics System Toolbox  SourceProductBaseCode=RO
  Mux : Mux  Inputs=5
  Terminator{,1..4} (5 alike) : Terminator
  param : Outport
  wires:
  Get Parameter/1 -> Mux/3
  Get Parameter1/1 -> Mux/4
  Get Parameter2/1 -> Mux/2
  Get Parameter4/1 -> Mux/5
  Get Parameter2/2 -> Terminator1/1
  Mux/1 -> param/1
  Get Parameter4/2 -> Terminator4/1
  Get Parameter/2 -> Terminator2/1
  Get Parameter1/2 -> Terminator3/1
  Get Parameter3/1 -> Mux/1
  Get Parameter3/2 -> Terminator/1

== system dx_hand_model_rai3/Pinky Finger/Pose Generator/Parametri Ring/Hand_written ==
  Antonio : Constant  Value=[ 8, 44.755952819297409619589520899781, 0, 1645979925414585/70368744177664, 0]
  Antonio Stimato : Constant  Value="[10.0000   46.0001    5.0000   17.9112         0]"
  Mano Domenico Stimata : Constant  Value="[9.5248   43.5033         0   10.2567   -1.6252]"
  Mano Legno : Constant  Value="[8   56   6    23 0]"
  Mano Legno Stimata : Constant  Value=[ 8, 60.637566881231091700096944861316, 0, 5166787254901141/281474976710656 0]
  Mano Legno Stimata1 : Constant  Value="[9.9977   51.1548    2.0668   25.1677         0]"
  Mano Legno1 : Constant  Value="[10.8169   54.9796    1.9601   28.8058]"
  Mano Max Reale : Constant  Value=[8 40 0 23 0]
  Mano Max Stimata : Constant  Value=[ 8, 48.37173324617629829549070114942, 0, 6626664510253941/281474976710656, 0]
  Mano Paolo Stimata : Constant  Value="[10.0000   46.0015    1.3696   13.2621         0]"
  Out2 : Outport
  wires:
  Antonio/1 -> Out2/1

== system dx_hand_model_rai3/Pinky Finger/Position-Force Architecture/Position Force Basic Architecture/f_gains//dist ==
  pre_dist : Inport
  Constant : Constant  Value=10  OutDataTypeStr=single
  Data Type Conversion1 : DataTypeConversion  OutDataTypeStr=single
  Data Type Conversion2 : DataTypeConversion  OutDataTypeStr=single
  Get Parameter3 : robotlib/Get Parameter  SourceLibraryInfo=This block requires Robotics System Toolbox  ParameterSource=Specify your own  ParameterName=/hand_exo/pinky/f_gains/dist  ParameterType=double  ParameterMaxArrayLength=16  ParameterInitialValue=10  SampleTime=update_param  ShowErrorCodeOutput=on  ModelName=dx_hand_model_rai3  BlockId=ParamGet_dx_hand_model_rai3_4700
      settings: SourceProductName=Robotics System Toolbox  SourceProductBaseCode=RO
  Manual Switch : ManualSwitch
  Product : Product
  Rate Transition : RateTransition
  post_dist : Outport
  wires:
  Get Parameter3/1 -> Rate Transition/1
  pre_dist/1 -> Product/2
  Product/1 -> Data Type Conversion1/1
  Data Type Conversion1/1 -> post_dist/1
  Rate Transition/1 -> Data Type Conversion2/1
  Constant/1 -> Manual Switch/2
  Data Type Conversion2/1 -> Manual Switch/1
  Manual Switch/1 -> Product/1

== system dx_hand_model_rai3/Pinky Finger/Position-Force Architecture/Position Force Basic Architecture/f_gains//prox ==
  pre_prox : Inport
  Constant : Constant  Value=-15  OutDataTypeStr=single
  Data Type Conversion1 : DataTypeConversion  OutDataTypeStr=single
  Data Type Conversion2 : DataTypeConversion  OutDataTypeStr=single
  Get Parameter3 : robotlib/Get Parameter  SourceLibraryInfo=This block requires Robotics System Toolbox  ParameterSource=Specify your own  ParameterName=/hand_exo/pinky/f_gains/prox  ParameterType=double  ParameterMaxArrayLength=16  ParameterInitialValue=-15  SampleTime=update_param  ShowErrorCodeOutput=on  ModelName=dx_hand_model_rai3  BlockId=ParamGet_dx_hand_model_rai3_4710
      settings: SourceProductName=Robotics System Toolbox  SourceProductBaseCode=RO
  Manual Switch : ManualSwitch
  Product : Product
  Rate Transition : RateTransition
  post_prox : Outport
  wires:
  Get Parameter3/1 -> Rate Transition/1
  pre_prox/1 -> Product/2
  Product/1 -> Data Type Conversion1/1
  Data Type Conversion1/1 -> post_prox/1
  Rate Transition/1 -> Data Type Conversion2/1
  Data Type Conversion2/1 -> Manual Switch/1
  Manual Switch/1 -> Product/1
  Constant/1 -> Manual Switch/2
